simulink model "task_B_All_mod"  (R2018a)
settings: Solver=ode45  StartTime=0.0  StopTime=70  RelTol=1e-3  EnableMultiTasking=on
values from neighbouring files (symbols this model uses):
  a0 = 8*lamda/(c*ro*(b-a)^2)    [task_A_scr.m]    (also in task_B_scr.m = 8*lamda/(3*c*ro*(b-a)^2); task_C_scr.m = 4*lamda*(2-A1-B1)/(c*ro*(b-a)^2))
  b0 = a0/2    [task_A_scr.m]    (also in task_B_scr.m)
  q_a = 500000    [task_B_scr.m]
  T_b = 400    [task_A_scr.m]    (also in task_B_scr.m = 350; task_C_scr.m = 300)
undefined symbols (not defined in the file or in its folder): a, b, lamda, T_0
settings Model: Creator=Yurii  LastModifiedBy=Master
settings DataIOCC: LimitDataPoints=on  SaveFormat=Array
settings OptimizationCC: LifeSpan=inf
settings DebuggingCC: UnderspecifiedInitializationDetection=Classic  MergeDetectMultiDrivingBlocksExec=none  SolverPrmCheckMsg=warning  SFUnexpectedBacktrackingDiag=warning  SFNoUnconditionalDefaultTransitionDiag=warning  SFExecutionAtInitializationDiag=none
settings HardwareCC: ProdBitPerPointer=32  ProdBitPerSizeT=32  ProdBitPerPtrDiffT=32  ProdLargestAtomicFloat=None  ProdIntDivRoundTo=Undefined  ProdEndianess=Unspecified  ProdWordSize=32  ProdHWDeviceType=32-bit Generic
settings ModelReferenceCC: PropagateSignalLabelsOutOfModel=off
settings CodeAppCC: StateflowObjectComments=on
settings GRTTargetCC: TargetLangStandard=C89/C90 (ANSI)  GeneratePreprocessorConditionals=Disable all
settings ConfigComp: CovMetricSettings=dw  CovHtmlReporting=on  CovSaveCumulativeToWorkspaceVar=on  CovSaveSingleToWorkspaceVar=on  CovExternalEMLEnable=off

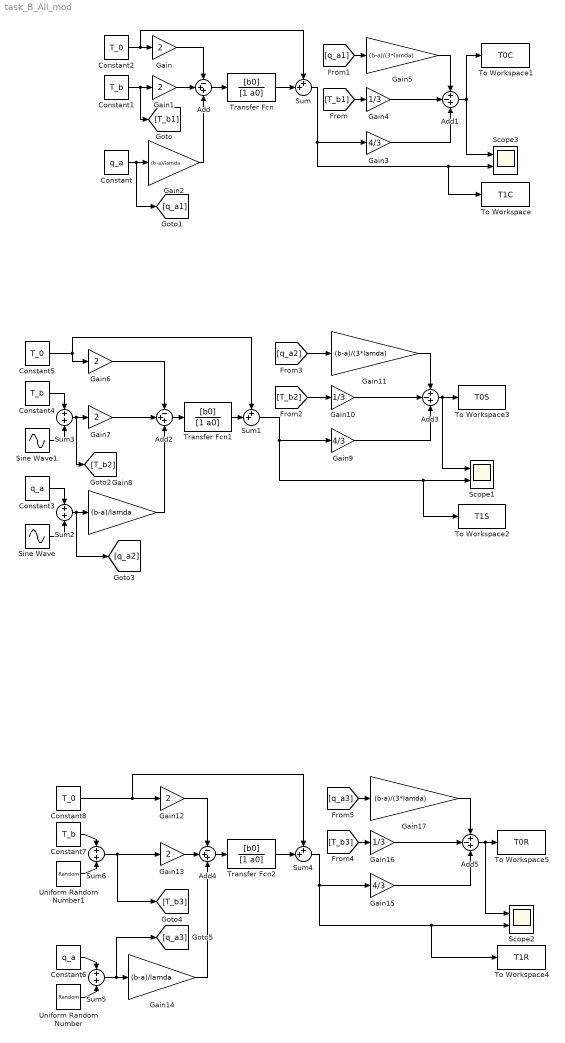
== system task_B_All_mod ==
  Add : Sum  Inputs=-++
  Add1 : Sum  Inputs=+-+
  Add2 : Sum  Inputs=-++
  Add3 : Sum  Inputs=+-+
  Add4 : Sum  Inputs=-++
  Add5 : Sum  Inputs=+-+
  Constant : Constant  Value=q_a
  Constant1 : Constant  Value=T_b
  Constant2 : Constant  Value=T_0
  Constant3 : Constant  Value=q_a
  Constant4 : Constant  Value=T_b
  Constant5 : Constant  Value=T_0
  Constant6 : Constant  Value=q_a
  Constant7 : Constant  Value=T_b
  Constant8 : Constant  Value=T_0
  Gain{,1,6..7,12..13} (6 alike) : Gain  Gain=2
  Gain10 : Gain  Gain=1/3
  Gain11 : Gain  Gain=(b-a)/(3*lamda)
  Gain14 : Gain  Gain=(b-a)/lamda
  Gain15 : Gain  Gain=4/3
  Gain16 : Gain  Gain=1/3
  Gain17 : Gain  Gain=(b-a)/(3*lamda)
  Gain2 : Gain  Gain=(b-a)/lamda
  Gain3 : Gain  Gain=4/3
  Gain4 : Gain  Gain=1/3
  Gain5 : Gain  Gain=(b-a)/(3*lamda)
  Gain8 : Gain  Gain=(b-a)/lamda
  Gain9 : Gain  Gain=4/3
  Scope1 : Scope  NumInputPorts=2
  Scope2 : Scope  NumInputPorts=2
  Scope3 : Scope  NumInputPorts=2
  Sine Wave : Sin  Amplitude=0.05*q_a  SampleTime=0
  Sine Wave1 : Sin  Amplitude=0.05*T_b  SampleTime=0
  Sum : Sum  Inputs=++|
  Sum1 : Sum  Inputs=++|
  Sum{2..3,5..6} (4 alike) : Sum  Inputs=+|+
  Sum4 : Sum  Inputs=++|
  To Workspace : ToWorkspace  VariableName=T1C  SaveFormat=Timeseries  SampleTime=-1
  To Workspace1 : ToWorkspace  VariableName=T0C  SaveFormat=Timeseries  SampleTime=-1
  To Workspace2 : ToWorkspace  VariableName=T1S  SaveFormat=Timeseries  SampleTime=-1
  To Workspace3 : ToWorkspace  VariableName=T0S  SaveFormat=Timeseries  SampleTime=-1
  To Workspace4 : ToWorkspace  VariableName=T1R  SaveFormat=Timeseries  SampleTime=-1
  To Workspace5 : ToWorkspace  VariableName=T0R  SaveFormat=Timeseries  SampleTime=-1
  Transfer Fcn : TransferFcn  Numerator=[b0]  Denominator=[1 a0]
  Transfer Fcn1 : TransferFcn  Numerator=[b0]  Denominator=[1 a0]
  Transfer Fcn2 : TransferFcn  Numerator=[b0]  Denominator=[1 a0]
  Uniform Random Number : UniformRandomNumber  Minimum=-0.05*q_a  Maximum=0.05*q_a  SampleTime=0.1
  Uniform Random Number1 : UniformRandomNumber  Minimum=-0.05*T_b  Maximum=0.05*T_b  SampleTime=0.1
  wires:
  Constant/1 -> [q_a1], Gain2/1
  Constant1/1 -> [T_b1], Gain1/1
  Constant2/1 -> Gain/1, Sum/1
  Gain/1 -> Add/1
  Add/1 -> Transfer Fcn/1
  Transfer Fcn/1 -> Sum/2
  Sum/1 -> Scope3/2, To Workspace/1, Gain3/1
  Gain1/1 -> Add/2
  Gain2/1 -> Add/3
  [T_b1] -> Gain4/1
  [q_a1] -> Gain5/1
  Gain4/1 -> Add1/2
  Gain5/1 -> Add1/1
  Gain3/1 -> Add1/3
  Add1/1 -> Scope3/1, To Workspace1/1
  Sine Wave1/1 -> Sum3/2
  Constant4/1 -> Sum3/1
  [T_b2] -> Gain10/1
  Sum2/1 -> [q_a2], Gain8/1
  Gain10/1 -> Add3/2
  Constant5/1 -> Sum1/1, Gain6/1
  Constant3/1 -> Sum2/1
  Gain6/1 -> Add2/1
  Gain8/1 -> Add2/3
  Gain9/1 -> Add3/3
  Gain11/1 -> Add3/1
  [q_a2] -> Gain11/1
  Sum3/1 -> [T_b2], Gain7/1
  Gain7/1 -> Add2/2
  Add3/1 -> Scope1/1, To Workspace3/1
  Sum1/1 -> Scope1/2, To Workspace2/1, Gain9/1
  Sine Wave/1 -> Sum2/2
  Transfer Fcn1/1 -> Sum1/2
  Add2/1 -> Transfer Fcn1/1
  Gain17/1 -> Add5/1
  Gain13/1 -> Add4/2
  Constant6/1 -> Sum5/1
  Constant7/1 -> Sum6/1
  Uniform Random Number1/1 -> Sum6/2
  Sum5/1 -> [q_a3], Gain14/1
  Transfer Fcn2/1 -> Sum4/2
  Add5/1 -> Scope2/1, To Workspace5/1
  Constant8/1 -> Gain12/1, Sum4/1
  Sum4/1 -> Scope2/2, To Workspace4/1, Gain15/1
  Uniform Random Number/1 -> Sum5/2
  Add4/1 -> Transfer Fcn2/1
  Sum6/1 -> [T_b3], Gain13/1
  Gain14/1 -> Add4/3
  Gain12/1 -> Add4/1
  [T_b3] -> Gain16/1
  Gain15/1 -> Add5/3
  Gain16/1 -> Add5/2
  [q_a3] -> Gain17/1
